simulink model "ClosedLoop"  (R2018b)
settings: Solver=VariableStepAuto  StartTime=0.0  StopTime=10  RelTol=1e-3
libraries: neural x533
(part 16 of 24)

== system ClosedLoop/Feed-Forward Neural Network/Layer 1/IW{1,1} ==
  "pd{1,1}" : Inport  PortDimensions=5
      mask Display: e = 0.06;c1 = [120 230 180]/255;c2 = ([120 230 180]+0)/(256+128);c3 = ([120 230 180]+128)/(256+128);patch([0 1 1 0],[0 0 1 1],c1);patch([0 1 1 1-e 1-e 0+e],[0 0 1 1-e 0+e 0+e],c2);patch([0 0 1 1-e 0+e 0+e],[0 1 1 1-e 1-e 0+e],c3);plot([0 1 1 0 0],[0 0 1 1 0]);
  "IW{1,1}(1,:)'" : Constant  Value=[0.777433677520860566545479741762392222881317138671875;0.73019317994989474396305695336195640265941619873046875;-0.69689232254614952299931474044569768011569976806640625;0.5351561132679254484401099034585058689117431640625;0.8471870111859789442831925043719820678234100341796875]
      mask Display: e = 0.06;c1 = [120 150 230]/255;c2 = ([120 150 230]+0)/383;c3 = ([120 150 230]+128)/383;patch([0 1 1 0],[0 0 1 1],c1);patch([0 1 1 1-e 1-e 0+e],[0 0 1 1-e 0+e 0+e],c2);patch([0 0 1 1-e 0+e 0+e],[0 1 1 1-e 1-e 0+e],c3);plot([0 1 1 0 0],[0 0 1 1 0]);disp('Weights');
  "IW{1,1}(10,:)'" : Constant  Value=[-0.08887973831498015286900482578857918269932270050048828125;-0.148128852319696802108950350884697400033473968505859375;0.489876132094335614564073466681293211877346038818359375;-0.004453902948160336737470910151159841916523873805999755859375;-0.36708303277551956877999828066094778478145599365234375]
      mask Display: e = 0.06;c1 = [120 150 230]/255;c2 = ([120 150 230]+0)/383;c3 = ([120 150 230]+128)/383;patch([0 1 1 0],[0 0 1 1],c1);patch([0 1 1 1-e 1-e 0+e],[0 0 1 1-e 0+e 0+e],c2);patch([0 0 1 1-e 0+e 0+e],[0 1 1 1-e 1-e 0+e],c3);plot([0 1 1 0 0],[0 0 1 1 0]);disp('Weights');
  "IW{1,1}(11,:)'" : Constant  Value=[0.257842561827505090121803732472471892833709716796875;0.2159497882699046578114376870871637947857379913330078125;-0.1732667109248870185300717139398329891264438629150390625;-0.229891953399321113948872152832336723804473876953125;-0.289081418236195986093406418149243108928203582763671875]
      mask Display: e = 0.06;c1 = [120 150 230]/255;c2 = ([120 150 230]+0)/383;c3 = ([120 150 230]+128)/383;patch([0 1 1 0],[0 0 1 1],c1);patch([0 1 1 1-e 1-e 0+e],[0 0 1 1-e 0+e 0+e],c2);patch([0 0 1 1-e 0+e 0+e],[0 1 1 1-e 1-e 0+e],c3);plot([0 1 1 0 0],[0 0 1 1 0]);disp('Weights');
  "IW{1,1}(12,:)'" : Constant  Value=[0.99297918861983658356251680743298493325710296630859375;-0.85768613628434042794879132998175919055938720703125;-0.1692019190082666157959323527393280528485774993896484375;-0.0360713330703844314850670116356923244893550872802734375;-0.82372546542318836326757036658818833529949188232421875]
      mask Display: e = 0.06;c1 = [120 150 230]/255;c2 = ([120 150 230]+0)/383;c3 = ([120 150 230]+128)/383;patch([0 1 1 0],[0 0 1 1],c1);patch([0 1 1 1-e 1-e 0+e],[0 0 1 1-e 0+e 0+e],c2);patch([0 0 1 1-e 0+e 0+e],[0 1 1 1-e 1-e 0+e],c3);plot([0 1 1 0 0],[0 0 1 1 0]);disp('Weights');
  "IW{1,1}(13,:)'" : Constant  Value=[-0.5601984423210086827538134457427076995372772216796875;0.8495448623663961473795325218816287815570831298828125;0.9142783166217982593337865182547830045223236083984375;-0.3151571944657833856950901463278569281101226806640625;-0.403790280453586003517330027534626424312591552734375]
      mask Display: e = 0.06;c1 = [120 150 230]/255;c2 = ([120 150 230]+0)/383;c3 = ([120 150 230]+128)/383;patch([0 1 1 0],[0 0 1 1],c1);patch([0 1 1 1-e 1-e 0+e],[0 0 1 1-e 0+e 0+e],c2);patch([0 0 1 1-e 0+e 0+e],[0 1 1 1-e 1-e 0+e],c3);plot([0 1 1 0 0],[0 0 1 1 0]);disp('Weights');
  "IW{1,1}(14,:)'" : Constant  Value=[-0.22742222534104128417453694055438973009586334228515625;0.287165266863248114237450181462918408215045928955078125;-0.2107887312575451865814812890675966627895832061767578125;0.384901355748308915405431207545916549861431121826171875;0.35264429343572889496982725177076645195484161376953125]
      mask Display: e = 0.06;c1 = [120 150 230]/255;c2 = ([120 150 230]+0)/383;c3 = ([120 150 230]+128)/383;patch([0 1 1 0],[0 0 1 1],c1);patch([0 1 1 1-e 1-e 0+e],[0 0 1 1-e 0+e 0+e],c2);patch([0 0 1 1-e 0+e 0+e],[0 1 1 1-e 1-e 0+e],c3);plot([0 1 1 0 0],[0 0 1 1 0]);disp('Weights');
  "IW{1,1}(15,:)'" : Constant  Value=[-0.4675162416237463869350676759495399892330169677734375;-0.791000664204850156835391317144967615604400634765625;0.203085187031351921405075700022280216217041015625;-0.2321122752203861328013090314925648272037506103515625;0.0023001892920386790564180046203546226024627685546875]
      mask Display: e = 0.06;c1 = [120 150 230]/255;c2 = ([120 150 230]+0)/383;c3 = ([120 150 230]+128)/383;patch([0 1 1 0],[0 0 1 1],c1);patch([0 1 1 1-e 1-e 0+e],[0 0 1 1-e 0+e 0+e],c2);patch([0 0 1 1-e 0+e 0+e],[0 1 1 1-e 1-e 0+e],c3);plot([0 1 1 0 0],[0 0 1 1 0]);disp('Weights');
  "IW{1,1}(16,:)'" : Constant  Value=[-0.370253147285887040940366432550945319235324859619140625;0.4026322235831856222176838855375535786151885986328125;0.454093022082059316613111832339200191199779510498046875;0.2183286697378135354785655408704769797623157501220703125;0.84167058255132121136199430111446417868137359619140625]
      mask Display: e = 0.06;c1 = [120 150 230]/255;c2 = ([120 150 230]+0)/383;c3 = ([120 150 230]+128)/383;patch([0 1 1 0],[0 0 1 1],c1);patch([0 1 1 1-e 1-e 0+e],[0 0 1 1-e 0+e 0+e],c2);patch([0 0 1 1-e 0+e 0+e],[0 1 1 1-e 1-e 0+e],c3);plot([0 1 1 0 0],[0 0 1 1 0]);disp('Weights');
  "IW{1,1}(17,:)'" : Constant  Value=[-0.6232209169783458069247217281372286379337310791015625;-0.208391342343335228548539816983975470066070556640625;0.357556683342926451274479404673911631107330322265625;-0.03813318521609776468039854080416262149810791015625;-0.8842941938241233312822942025377415120601654052734375]
      mask Display: e = 0.06;c1 = [120 150 230]/255;c2 = ([120 150 230]+0)/383;c3 = ([120 150 230]+128)/383;patch([0 1 1 0],[0 0 1 1],c1);patch([0 1 1 1-e 1-e 0+e],[0 0 1 1-e 0+e 0+e],c2);patch([0 0 1 1-e 0+e 0+e],[0 1 1 1-e 1-e 0+e],c3);plot([0 1 1 0 0],[0 0 1 1 0]);disp('Weights');
  "IW{1,1}(18,:)'" : Constant  Value=[-0.73987952043528881773681860067881643772125244140625;-0.82018478772733593995525325226481072604656219482421875;-0.3600533958394851463680197412031702697277069091796875;0.3501309983575382478449000700493343174457550048828125;-0.008329197715858167871960660022523370571434497833251953125]
      mask Display: e = 0.06;c1 = [120 150 230]/255;c2 = ([120 150 230]+0)/383;c3 = ([120 150 230]+128)/383;patch([0 1 1 0],[0 0 1 1],c1);patch([0 1 1 1-e 1-e 0+e],[0 0 1 1-e 0+e 0+e],c2);patch([0 0 1 1-e 0+e 0+e],[0 1 1 1-e 1-e 0+e],c3);plot([0 1 1 0 0],[0 0 1 1 0]);disp('Weights');
  "IW{1,1}(19,:)'" : Constant  Value=[-0.189399706316041804843308682393399067223072052001953125;-0.575158414122049155281501953140832483768463134765625;-0.64617497840545379261811831383965909481048583984375;0.61003694509276495949734453461132943630218505859375;-0.01759269567811309886717907602360355667769908905029296875]
      mask Display: e = 0.06;c1 = [120 150 230]/255;c2 = ([120 150 230]+0)/383;c3 = ([120 150 230]+128)/383;patch([0 1 1 0],[0 0 1 1],c1);patch([0 1 1 1-e 1-e 0+e],[0 0 1 1-e 0+e 0+e],c2);patch([0 0 1 1-e 0+e 0+e],[0 1 1 1-e 1-e 0+e],c3);plot([0 1 1 0 0],[0 0 1 1 0]);disp('Weights');
  "IW{1,1}(2,:)'" : Constant  Value=[0.63621458796631624732498266894253902137279510498046875;0.0583211436143939165877014829675317741930484771728515625;0.2549619279325689991111403287504799664020538330078125;-0.06918783634941839955079245783053920604288578033447265625;-0.52938238600419096346882952275336720049381256103515625]
      mask Display: e = 0.06;c1 = [120 150 230]/255;c2 = ([120 150 230]+0)/383;c3 = ([120 150 230]+128)/383;patch([0 1 1 0],[0 0 1 1],c1);patch([0 1 1 1-e 1-e 0+e],[0 0 1 1-e 0+e 0+e],c2);patch([0 0 1 1-e 0+e 0+e],[0 1 1 1-e 1-e 0+e],c3);plot([0 1 1 0 0],[0 0 1 1 0]);disp('Weights');
  "IW{1,1}(20,:)'" : Constant  Value=[-0.320099217953699832772684885640046559274196624755859375;-0.493413713263920694629405261366628110408782958984375;-0.258427516551161529090308022205135785043239593505859375;0.038020508091600242750462967933344771154224872589111328125;0.040457121285289963930065226804799749515950679779052734375]
      mask Display: e = 0.06;c1 = [120 150 230]/255;c2 = ([120 150 230]+0)/383;c3 = ([120 150 230]+128)/383;patch([0 1 1 0],[0 0 1 1],c1);patch([0 1 1 1-e 1-e 0+e],[0 0 1 1-e 0+e 0+e],c2);patch([0 0 1 1-e 0+e 0+e],[0 1 1 1-e 1-e 0+e],c3);plot([0 1 1 0 0],[0 0 1 1 0]);disp('Weights');
  "IW{1,1}(3,:)'" : Constant  Value=[-0.55562414003558036057484059710986912250518798828125;0.828270336283832175894303873064927756786346435546875;0.50830517043565492940615513361990451812744140625;-0.070744457945359773276550185983069241046905517578125;0.746438680345809846272686627344228327274322509765625]
      mask Display: e = 0.06;c1 = [120 150 230]/255;c2 = ([120 150 230]+0)/383;c3 = ([120 150 230]+128)/383;patch([0 1 1 0],[0 0 1 1],c1);patch([0 1 1 1-e 1-e 0+e],[0 0 1 1-e 0+e 0+e],c2);patch([0 0 1 1-e 0+e 0+e],[0 1 1 1-e 1-e 0+e],c3);plot([0 1 1 0 0],[0 0 1 1 0]);disp('Weights');
  "IW{1,1}(4,:)'" : Constant  Value=[0.75580233193780987921428504705545492470264434814453125;0.9364857196000182515405185768031515181064605712890625;-0.00704463179962803477673904950506766908802092075347900390625;-0.121740150618717624109166308699059300124645233154296875;-0.5242409013589768296270676728454418480396270751953125]
      mask Display: e = 0.06;c1 = [120 150 230]/255;c2 = ([120 150 230]+0)/383;c3 = ([120 150 230]+128)/383;patch([0 1 1 0],[0 0 1 1],c1);patch([0 1 1 1-e 1-e 0+e],[0 0 1 1-e 0+e 0+e],c2);patch([0 0 1 1-e 0+e 0+e],[0 1 1 1-e 1-e 0+e],c3);plot([0 1 1 0 0],[0 0 1 1 0]);disp('Weights');
  "IW{1,1}(5,:)'" : Constant  Value=[-1.233281510246877044068014583899639546871185302734375;0.1540174951845404149874951826859614811837673187255859375;0.3254058096269802913269586497335694730281829833984375;0.52623232596991720289025806778226979076862335205078125;0.15639372788910943512519224896095693111419677734375]
      mask Display: e = 0.06;c1 = [120 150 230]/255;c2 = ([120 150 230]+0)/383;c3 = ([120 150 230]+128)/383;patch([0 1 1 0],[0 0 1 1],c1);patch([0 1 1 1-e 1-e 0+e],[0 0 1 1-e 0+e 0+e],c2);patch([0 0 1 1-e 0+e 0+e],[0 1 1 1-e 1-e 0+e],c3);plot([0 1 1 0 0],[0 0 1 1 0]);disp('Weights');
  "IW{1,1}(6,:)'" : Constant  Value=[-0.2123808527301400961295740899004158563911914825439453125;-0.7650063601999883555748738217516802251338958740234375;0.2036265237720711607227741524184239096939563751220703125;0.2350543570458159259306540889156167395412921905517578125;-0.61247535013271681147983827031566761434078216552734375]
      mask Display: e = 0.06;c1 = [120 150 230]/255;c2 = ([120 150 230]+0)/383;c3 = ([120 150 230]+128)/383;patch([0 1 1 0],[0 0 1 1],c1);patch([0 1 1 1-e 1-e 0+e],[0 0 1 1-e 0+e 0+e],c2);patch([0 0 1 1-e 0+e 0+e],[0 1 1 1-e 1-e 0+e],c3);plot([0 1 1 0 0],[0 0 1 1 0]);disp('Weights');
  "IW{1,1}(7,:)'" : Constant  Value=[-0.145913693400883115458555039367638528347015380859375;0.85518026859664908467806299086078070104122161865234375;0.62282664130440179572900660787126980721950531005859375;0.2429637230793593172251121359295211732387542724609375;0.43881248529995386942204049773863516747951507568359375]
      mask Display: e = 0.06;c1 = [120 150 230]/255;c2 = ([120 150 230]+0)/383;c3 = ([120 150 230]+128)/383;patch([0 1 1 0],[0 0 1 1],c1);patch([0 1 1 1-e 1-e 0+e],[0 0 1 1-e 0+e 0+e],c2);patch([0 0 1 1-e 0+e 0+e],[0 1 1 1-e 1-e 0+e],c3);plot([0 1 1 0 0],[0 0 1 1 0]);disp('Weights');
  "IW{1,1}(8,:)'" : Constant  Value=[-0.19941423223278942344904862693510949611663818359375;0.1871215449623158111336351794307120144367218017578125;0.2685564059652356672103223900194279849529266357421875;-0.677958190830524554115754654048942029476165771484375;-0.6415809984175366853520472432137466967105865478515625]
      mask Display: e = 0.06;c1 = [120 150 230]/255;c2 = ([120 150 230]+0)/383;c3 = ([120 150 230]+128)/383;patch([0 1 1 0],[0 0 1 1],c1);patch([0 1 1 1-e 1-e 0+e],[0 0 1 1-e 0+e 0+e],c2);patch([0 0 1 1-e 0+e 0+e],[0 1 1 1-e 1-e 0+e],c3);plot([0 1 1 0 0],[0 0 1 1 0]);disp('Weights');
  "IW{1,1}(9,:)'" : Constant  Value=[-0.7761547121882117483693264148314483463764190673828125;0.767230609849536282496273997821845114231109619140625;0.20091122506164094119185392628423869609832763671875;-0.1352463461126560684277819746057502925395965576171875;-0.669215506292098805118939708336256444454193115234375]
      mask Display: e = 0.06;c1 = [120 150 230]/255;c2 = ([120 150 230]+0)/383;c3 = ([120 150 230]+128)/383;patch([0 1 1 0],[0 0 1 1],c1);patch([0 1 1 1-e 1-e 0+e],[0 0 1 1-e 0+e 0+e],c2);patch([0 0 1 1-e 0+e 0+e],[0 1 1 1-e 1-e 0+e],c3);plot([0 1 1 0 0],[0 0 1 1 0]);disp('Weights');
  Mux : Mux  Inputs=20
      mask Display: e = 0.06;c1 = [120 150 230]/255;c2 = ([120 150 230]+0)/383;c3 = ([120 150 230]+128)/383;patch([0 1 1 0],[0 0 1 1],c1);patch([0 1 1 1-e 1-e 0+e],[0 0 1 1-e 0+e 0+e],c2);patch([0 0 1 1-e 0+e 0+e],[0 1 1 1-e 1-e 0+e],c3);plot([0 1 1 0 0],[0 0 1 1 0]);disp('Mux');
  dotprod{1..20} (20 alike) : neural/Weight Functions/dotprod
  "iz{1,1}" : Outport
      mask Display: e = 0.06;c1 = [120 230 180]/255;c2 = ([120 230 180]+0)/(256+128);c3 = ([120 230 180]+128)/(256+128);patch([0 1 1 0],[0 0 1 1],c1);patch([0 1 1 1-e 1-e 0+e],[0 0 1 1-e 0+e 0+e],c2);patch([0 0 1 1-e 0+e 0+e],[0 1 1 1-e 1-e 0+e],c3);plot([0 1 1 0 0],[0 0 1 1 0]);
  wires:
  Mux/1 -> "iz{1,1}"/1
  dotprod20/1 -> Mux/20
  "IW{1,1}(20,:)'"/1 -> dotprod20/1
  dotprod19/1 -> Mux/19
  "IW{1,1}(19,:)'"/1 -> dotprod19/1
  dotprod18/1 -> Mux/18
  "IW{1,1}(18,:)'"/1 -> dotprod18/1
  dotprod17/1 -> Mux/17
  "IW{1,1}(17,:)'"/1 -> dotprod17/1
  dotprod16/1 -> Mux/16
  "IW{1,1}(16,:)'"/1 -> dotprod16/1
  dotprod15/1 -> Mux/15
  "IW{1,1}(15,:)'"/1 -> dotprod15/1
  dotprod14/1 -> Mux/14
  "IW{1,1}(14,:)'"/1 -> dotprod14/1
  dotprod13/1 -> Mux/13
  "IW{1,1}(13,:)'"/1 -> dotprod13/1
  dotprod12/1 -> Mux/12
  "IW{1,1}(12,:)'"/1 -> dotprod12/1
  dotprod11/1 -> Mux/11
  "IW{1,1}(11,:)'"/1 -> dotprod11/1
  dotprod10/1 -> Mux/10
  "IW{1,1}(10,:)'"/1 -> dotprod10/1
  dotprod9/1 -> Mux/9
  "IW{1,1}(9,:)'"/1 -> dotprod9/1
  dotprod8/1 -> Mux/8
  "IW{1,1}(8,:)'"/1 -> dotprod8/1
  dotprod7/1 -> Mux/7
  "IW{1,1}(7,:)'"/1 -> dotprod7/1
  dotprod6/1 -> Mux/6
  "IW{1,1}(6,:)'"/1 -> dotprod6/1
  dotprod5/1 -> Mux/5
  "IW{1,1}(5,:)'"/1 -> dotprod5/1
  dotprod4/1 -> Mux/4
  "IW{1,1}(4,:)'"/1 -> dotprod4/1
  dotprod3/1 -> Mux/3
  "IW{1,1}(3,:)'"/1 -> dotprod3/1
  dotprod2/1 -> Mux/2
  "IW{1,1}(2,:)'"/1 -> dotprod2/1
  dotprod1/1 -> Mux/1
  "pd{1,1}"/1 -> dotprod20/2, dotprod19/2, dotprod18/2, dotprod17/2, dotprod16/2, dotprod15/2, dotprod14/2, dotprod13/2, dotprod12/2, dotprod11/2, dotprod10/2, dotprod9/2, dotprod8/2, dotprod7/2, dotprod6/2, dotprod5/2, dotprod4/2, dotprod3/2, dotprod2/2, dotprod1/2
  "IW{1,1}(1,:)'"/1 -> dotprod1/1

== system ClosedLoop/Feed-Forward Neural Network/Layer 10/Delays 1 ==
  "p{10}" : Inport  PortDimensions=20
      mask Display: e = 0.06;c1 = [120 230 180]/255;c2 = ([120 230 180]+0)/(256+128);c3 = ([120 230 180]+128)/(256+128);patch([0 1 1 0],[0 0 1 1],c1);patch([0 1 1 1-e 1-e 0+e],[0 0 1 1-e 0+e 0+e],c2);patch([0 0 1 1-e 0+e 0+e],[0 1 1 1-e 1-e 0+e],c3);plot([0 1 1 0 0],[0 0 1 1 0]);
  mux : Mux  Inputs=1
      mask Display: e = 0.06;c1 = [120 150 230]/255;c2 = ([120 150 230]+0)/383;c3 = ([120 150 230]+128)/383;patch([0 1 1 0],[0 0 1 1],c1);patch([0 1 1 1-e 1-e 0+e],[0 0 1 1-e 0+e 0+e],c2);patch([0 0 1 1-e 0+e 0+e],[0 1 1 1-e 1-e 0+e],c3);plot([0 1 1 0 0],[0 0 1 1 0]);disp('Mux')
  "pd{10,9}" : Outport
      mask Display: e = 0.06;c1 = [120 230 180]/255;c2 = ([120 230 180]+0)/(256+128);c3 = ([120 230 180]+128)/(256+128);patch([0 1 1 0],[0 0 1 1],c1);patch([0 1 1 1-e 1-e 0+e],[0 0 1 1-e 0+e 0+e],c2);patch([0 0 1 1-e 0+e 0+e],[0 1 1 1-e 1-e 0+e],c3);plot([0 1 1 0 0],[0 0 1 1 0]);
  wires:
  mux/1 -> "pd{10,9}"/1
  "p{10}"/1 -> mux/1

== system ClosedLoop/Feed-Forward Neural Network/Layer 10/LW{10,9} ==
  "ad{10,9}" : Inport  PortDimensions=20
      mask Display: e = 0.06;c1 = [120 230 180]/255;c2 = ([120 230 180]+0)/(256+128);c3 = ([120 230 180]+128)/(256+128);patch([0 1 1 0],[0 0 1 1],c1);patch([0 1 1 1-e 1-e 0+e],[0 0 1 1-e 0+e 0+e],c2);patch([0 0 1 1-e 0+e 0+e],[0 1 1 1-e 1-e 0+e],c3);plot([0 1 1 0 0],[0 0 1 1 0]);
  "IW{10,9}(1,:)'" : Constant  Value=[0.5466415304082350434811132799950428307056427001953125;-0.8271711330800453065847932521137408912181854248046875;0.621717062498548411753063192008994519710540771484375;-0.7617361424174025064104398552444763481616973876953125;0.323400873829868817921351364930160343647003173828125;0.5870808725143337181151537151890806853771209716796875;0.331754437350670006168229519971646368503570556640625;-0.81908419253871667109478948987089097499847412109375;0.8565616368669726199414071743376553058624267578125;0.706184991822760732560482210828922688961029052734375;-0.450365553497307669061910928576253354549407958984375;0.161786684402280389605266464059241116046905517578125;0.03591585902579108591226031421683728694915771484375;0.6471253790508237901946131387376226484775543212890625;-0.941846360469744237065015113330446183681488037109375;0.7218375932220528756744215570506639778614044189453125;0.8760431144644991174885717555298469960689544677734375;-0.5388868782146196689808448354597203433513641357421875;-0.0040941045081634985791652070474810898303985595703125;-0.9809642025486418059898596766288392245769500732421875]
      mask Display: e = 0.06;c1 = [120 150 230]/255;c2 = ([120 150 230]+0)/383;c3 = ([120 150 230]+128)/383;patch([0 1 1 0],[0 0 1 1],c1);patch([0 1 1 1-e 1-e 0+e],[0 0 1 1-e 0+e 0+e],c2);patch([0 0 1 1-e 0+e 0+e],[0 1 1 1-e 1-e 0+e],c3);plot([0 1 1 0 0],[0 0 1 1 0]);disp('weights');
  "IW{10,9}(10,:)'" : Constant  Value=[0.189578467104812631305321701802313327789306640625;-0.1971505451331568015138628879867610521614551544189453125;-0.0938551633204507407270966723444871604442596435546875;-0.0355861505184178472660505576641298830509185791015625;0.3106286001380731409682312005315907299518585205078125;-0.54752969328460177056427937714033760130405426025390625;-0.457848112424283471000308054499328136444091796875;0.066724722426169780220561733585782349109649658203125;0.3399176553675749001826034145778976380825042724609375;1.007552250911837976588003584765829145908355712890625;0.265730037797317464320911994946072809398174285888671875;-0.897550681116356496858088576118461787700653076171875;0.8924950068454950979912609909661114215850830078125;-0.734025961733759668703669376554898917675018310546875;0.30825870376673292216906929752440191805362701416015625;0.6367403979295145344252659924677573144435882568359375;0.9993387589299149720289960896479897201061248779296875;0.72728658684421232383243705044151283800601959228515625;-0.006671055503067472615408295411043582134880125522613525390625;0.53220228209855668932704020335222594439983367919921875]
      mask Display: e = 0.06;c1 = [120 150 230]/255;c2 = ([120 150 230]+0)/383;c3 = ([120 150 230]+128)/383;patch([0 1 1 0],[0 0 1 1],c1);patch([0 1 1 1-e 1-e 0+e],[0 0 1 1-e 0+e 0+e],c2);patch([0 0 1 1-e 0+e 0+e],[0 1 1 1-e 1-e 0+e],c3);plot([0 1 1 0 0],[0 0 1 1 0]);disp('weights');
  "IW{10,9}(11,:)'" : Constant  Value=[-0.4022891319285617495182805214426480233669281005859375;-0.684681661104177496923739454359747469425201416015625;-0.210482527346528502931732873548753559589385986328125;-0.009164173785581652964538079686462879180908203125;0.1336869968563314525766827500774525105953216552734375;-0.8154908488996941429149956093169748783111572265625;-0.7225052276356740410534484908566810190677642822265625;0.0533294738522041011918872754904441535472869873046875;0.59118399932295506715718147461302578449249267578125;0.5589665429530852325257228585542179644107818603515625;-0.260620748059805951157841263921000063419342041015625;-0.609699818746113120226937098777852952480316162109375;-0.17887626676285517390851964592002332210540771484375;-0.915665165190061802746868124813772737979888916015625;-0.2142521711594704836301161776646040380001068115234375;-0.279113013475847271394059134763665497303009033203125;-0.7416473991930951914497427424066700041294097900390625;-0.6497481904034076993781354758539237082004547119140625;-0.3051031869474079005755129401222802698612213134765625;0.6723350544936492756420420846552588045597076416015625]
      mask Display: e = 0.06;c1 = [120 150 230]/255;c2 = ([120 150 230]+0)/383;c3 = ([120 150 230]+128)/383;patch([0 1 1 0],[0 0 1 1],c1);patch([0 1 1 1-e 1-e 0+e],[0 0 1 1-e 0+e 0+e],c2);patch([0 0 1 1-e 0+e 0+e],[0 1 1 1-e 1-e 0+e],c3);plot([0 1 1 0 0],[0 0 1 1 0]);disp('weights');
  "IW{10,9}(12,:)'" : Constant  Value=[0.472535423523304742854378446281771175563335418701171875;-0.11729833819846562092958919265583972446620464324951171875;0.923190603308829960127468439168296754360198974609375;-0.37303267056098388110285668517462909221649169921875;-0.99375627128259669262888564844615757465362548828125;-0.482768672816777044687341913231648504734039306640625;-0.62074958062280927162390753437648527324199676513671875;0.30989821754524171648625952002475969493389129638671875;-0.4549131499265310907276216312311589717864990234375;0.991655015662607386417448651627637445926666259765625;-0.29993544946830674735593902369146235287189483642578125;-0.32489154519676832766350571546354331076145172119140625;-0.9793327969276492961370195189374499022960662841796875;-0.1979220780648585087391211345675401389598846435546875;0.2415191975738621987801479917834512889385223388671875;0.003048136298864800863839263911359012126922607421875;-0.4132587115501944463602512769284658133983612060546875;0.74981073939471365452646978155826218426227569580078125;0.544121005652982159261910055647604167461395263671875;0.23469808525191437897916557631106115877628326416015625]
      mask Display: e = 0.06;c1 = [120 150 230]/255;c2 = ([120 150 230]+0)/383;c3 = ([120 150 230]+128)/383;patch([0 1 1 0],[0 0 1 1],c1);patch([0 1 1 1-e 1-e 0+e],[0 0 1 1-e 0+e 0+e],c2);patch([0 0 1 1-e 0+e 0+e],[0 1 1 1-e 1-e 0+e],c3);plot([0 1 1 0 0],[0 0 1 1 0]);disp('weights');
  "IW{10,9}(13,:)'" : Constant  Value=[-0.2790275991646777864474415764561854302883148193359375;0.1921087329921764563778197043575346469879150390625;-0.9836433950387455382724510855041444301605224609375;-0.3529980607903995259988505495130084455013275146484375;0.3027029619324619336140358427655883133411407470703125;0.805139324920179699773825632291845977306365966796875;-0.0121052133967480823883988705347292125225067138671875;0.293128861832891995931049677892588078975677490234375;-0.4321697413435654500091231966507621109485626220703125;-0.02489408541289872545121397706679999828338623046875;-0.117315079294827651068544582813046872615814208984375;0.2856668033102902626296781818382441997528076171875;-0.3798620054401198320448429512907750904560089111328125;0.1914153748986400227494186765397898852825164794921875;-0.500452529632526843528239623992703855037689208984375;0.4953482368724262396852964229765348136425018310546875;-0.0462412526256865685780894636991433799266815185546875;-0.4407344712191016977698154732934199273586273193359375;-0.42942652906107259269674614188261330127716064453125;-0.9986097920558434370974509874940849840641021728515625]
      mask Display: e = 0.06;c1 = [120 150 230]/255;c2 = ([120 150 230]+0)/383;c3 = ([120 150 230]+128)/383;patch([0 1 1 0],[0 0 1 1],c1);patch([0 1 1 1-e 1-e 0+e],[0 0 1 1-e 0+e 0+e],c2);patch([0 0 1 1-e 0+e 0+e],[0 1 1 1-e 1-e 0+e],c3);plot([0 1 1 0 0],[0 0 1 1 0]);disp('weights');
  "IW{10,9}(14,:)'" : Constant  Value=[0.4369190502101643058807667330256663262844085693359375;-0.355337007376919533641057569184340536594390869140625;-0.2031226207170384601141677194391377270221710205078125;0.8182026275036318185840400474262423813343048095703125;-0.3658053117802866349705936954705975949764251708984375;-0.565304022594878663454665002063848078250885009765625;-0.8268329782883065970366942565306089818477630615234375;-0.6163385354199117927009865525178611278533935546875;0.4345114997214183372165052787750028073787689208984375;-0.7440346798558070684492804502951912581920623779296875;0.0322476965290927619633976064505986869335174560546875;-0.565192144773778437638611649163067340850830078125;-0.689586324724370314243060420267283916473388671875;0.8393585927691102899217412414145655930042266845703125;0.4546934662228012680174060733406804502010345458984375;0.6636997613296118370129761387943290174007415771484375;-0.740835135518632892370760600897483527660369873046875;0.6989520026872793057037824837607331573963165283203125;0.6487934190964834701986774234683252871036529541015625;-0.497449739803909718460772637627087533473968505859375]
      mask Display: e = 0.06;c1 = [120 150 230]/255;c2 = ([120 150 230]+0)/383;c3 = ([120 150 230]+128)/383;patch([0 1 1 0],[0 0 1 1],c1);patch([0 1 1 1-e 1-e 0+e],[0 0 1 1-e 0+e 0+e],c2);patch([0 0 1 1-e 0+e 0+e],[0 1 1 1-e 1-e 0+e],c3);plot([0 1 1 0 0],[0 0 1 1 0]);disp('weights');
  "IW{10,9}(15,:)'" : Constant  Value=[0.81888617750407999285044979842496104538440704345703125;0.5025381956551642215202946317731402814388275146484375;-0.0244554521771054300671721648541279137134552001953125;-0.0993267520517020496839677434763871133327484130859375;-0.468132325571704033251307919272221624851226806640625;-0.09717765831892821726256670444854535162448883056640625;0.98966986014234514801302111663972027599811553955078125;0.7609751275066820586090443612192757427692413330078125;-0.6307257641354617749840372198377735912799835205078125;-0.1676228780207849045069679050357080996036529541015625;-0.3440258172026455785186271896236576139926910400390625;-0.7504227920973811638560846404288895428180694580078125;0.9881650804532176035621660048491321504116058349609375;-0.4124483755117100969300736323930323123931884765625;-0.49281764969508190521452206667163409292697906494140625;-0.2110580359176890130612491702777333557605743408203125;-0.5437530697986987515690771033405326306819915771484375;0.3556834622381674915203575437772087752819061279296875;-0.5514986314494745300862632575444877147674560546875;-0.1793520366655853293114120106110931374132633209228515625]
      mask Display: e = 0.06;c1 = [120 150 230]/255;c2 = ([120 150 230]+0)/383;c3 = ([120 150 230]+128)/383;patch([0 1 1 0],[0 0 1 1],c1);patch([0 1 1 1-e 1-e 0+e],[0 0 1 1-e 0+e 0+e],c2);patch([0 0 1 1-e 0+e 0+e],[0 1 1 1-e 1-e 0+e],c3);plot([0 1 1 0 0],[0 0 1 1 0]);disp('weights');
  "IW{10,9}(16,:)'" : Constant  Value=[-0.807261281547004383440935271210037171840667724609375;-0.69747664444503654213036725195706821978092193603515625;0.2362735258440535890400724383653141558170318603515625;0.4972716005811157469196359670604579150676727294921875;-0.0791035934022248365948826176463626325130462646484375;0.82826415173932266267087243249989114701747894287109375;-0.7461955501513630739651716794469393789768218994140625;-0.570484902244871694421135543962009251117706298828125;0.66740671729979794690734706819057464599609375;0.4379669677018591666950442231609486043453216552734375;-0.067320615611759115903822703330661170184612274169921875;0.92242108976409731280199366665328852832317352294921875;-0.0995215907740083505217398851527832448482513427734375;0.0900786848374106607906242061289958655834197998046875;-0.62719102872585763552848447943688370287418365478515625;-0.806727306236569408071090947487391531467437744140625;-0.63785591144042452782514374121092259883880615234375;-0.518744383210614667945037581375800073146820068359375;0.72428274486928712061484247897169552743434906005859375;-0.04536905795470470847963184723994345404207706451416015625]
      mask Display: e = 0.06;c1 = [120 150 230]/255;c2 = ([120 150 230]+0)/383;c3 = ([120 150 230]+128)/383;patch([0 1 1 0],[0 0 1 1],c1);patch([0 1 1 1-e 1-e 0+e],[0 0 1 1-e 0+e 0+e],c2);patch([0 0 1 1-e 0+e 0+e],[0 1 1 1-e 1-e 0+e],c3);plot([0 1 1 0 0],[0 0 1 1 0]);disp('weights');
  "IW{10,9}(17,:)'" : Constant  Value=[-0.079824662453312489329704249030328355729579925537109375;-0.50863162741843892522553005619556643068790435791015625;-0.8599800118631446554928743353229947388172149658203125;-0.6294933410241403404228321960545144975185394287109375;0.2463218798189050762204033162561245262622833251953125;-0.61285062671762446928624967767973430454730987548828125;-0.6803704001432462344922669217339716851711273193359375;-0.1774127237379981014697705177241005003452301025390625;-0.660669974241251178881384475971572101116180419921875;0.343070582710990279462492935635964386165142059326171875;-0.98323676721291730640217565451166592538356781005859375;-0.59245292930485338178669962871936149895191192626953125;0.0904365751746156742996163302450440824031829833984375;0.5633635565556909252649120389833115041255950927734375;-0.40518767328097304858403049365733750164508819580078125;-0.4692167703492871044801404423196800053119659423828125;0.3440311556339554766026367360609583556652069091796875;0.957117910618051848103959855507127940654754638671875;0.843549532473236052254605965572409331798553466796875;0.7310783118291774851371656041010282933712005615234375]
      mask Display: e = 0.06;c1 = [120 150 230]/255;c2 = ([120 150 230]+0)/383;c3 = ([120 150 230]+128)/383;patch([0 1 1 0],[0 0 1 1],c1);patch([0 1 1 1-e 1-e 0+e],[0 0 1 1-e 0+e 0+e],c2);patch([0 0 1 1-e 0+e 0+e],[0 1 1 1-e 1-e 0+e],c3);plot([0 1 1 0 0],[0 0 1 1 0]);disp('weights');
  "IW{10,9}(18,:)'" : Constant  Value=[-0.741994973924807066367748120683245360851287841796875;0.76531031300398344452418086802936159074306488037109375;-0.7146241606467922391487945787957869470119476318359375;-0.830155959148634270405864299391396343708038330078125;0.603706861411432260666742877219803631305694580078125;-0.1606720355925517207396069352398626506328582763671875;0.48859267651597704240629127525608055293560028076171875;-0.53859492966335509311903706475277431309223175048828125;0.906531353405531259426197721040807664394378662109375;0.7759681652601961854287537789787165820598602294921875;-0.6899583681930383516345273164915852248668670654296875;0.892110625991080041785608045756816864013671875;-0.4753364439368537031072037279955111443996429443359375;-0.3452009165545935065466665037092752754688262939453125;-0.418831082050324543519792541701463051140308380126953125;0.5838900251042142830470993430935777723789215087890625;-0.3484303194405888870477383534307591617107391357421875;-0.498105927839950890501086178119294345378875732421875;-0.607485742647509763258995008072815835475921630859375;-0.86925862322098990109253691116464324295520782470703125]
      mask Display: e = 0.06;c1 = [120 150 230]/255;c2 = ([120 150 230]+0)/383;c3 = ([120 150 230]+128)/383;patch([0 1 1 0],[0 0 1 1],c1);patch([0 1 1 1-e 1-e 0+e],[0 0 1 1-e 0+e 0+e],c2);patch([0 0 1 1-e 0+e 0+e],[0 1 1 1-e 1-e 0+e],c3);plot([0 1 1 0 0],[0 0 1 1 0]);disp('weights');
  "IW{10,9}(19,:)'" : Constant  Value=[0.38736835788324730511789084630436263978481292724609375;0.52891329205685211345411289585172198712825775146484375;0.3084532647244804248742866548127494752407073974609375;-0.5859415921437653995695882258587516844272613525390625;0.1223282385631441204765224028960801661014556884765625;0.2590331905913878518532555972342379391193389892578125;0.2544295394265023713131768090534023940563201904296875;-0.3702353880002842156926590178045444190502166748046875;0.4450960903678173874453705138876102864742279052734375;0.426338109566266776351284306656452827155590057373046875;-0.270300401170748993973091955922427587211132049560546875;0.32578454574266169085916544645442627370357513427734375;0.76508246916542699267438365495763719081878662109375;-0.8094744632637753678494618725380860269069671630859375;-0.77472824799972894727062566744280047714710235595703125;0.873721485200615877175778223318047821521759033203125;0.5811750549824659106690205589984543621540069580078125;0.25099601908891866486328581231646239757537841796875;-0.88025669091856995063238855436793528497219085693359375;-0.23714177163528316061302803063881583511829376220703125]
      mask Display: e = 0.06;c1 = [120 150 230]/255;c2 = ([120 150 230]+0)/383;c3 = ([120 150 230]+128)/383;patch([0 1 1 0],[0 0 1 1],c1);patch([0 1 1 1-e 1-e 0+e],[0 0 1 1-e 0+e 0+e],c2);patch([0 0 1 1-e 0+e 0+e],[0 1 1 1-e 1-e 0+e],c3);plot([0 1 1 0 0],[0 0 1 1 0]);disp('weights');
  "IW{10,9}(2,:)'" : Constant  Value=[0.31123060134378077723482647343189455568790435791015625;-0.11598795207237037885317221252989838831126689910888671875;-0.9031465636276241326640956685878336429595947265625;-0.9137257980716524397024613790563307702541351318359375;0.878426312741913850601349622593261301517486572265625;-0.46316276823649926708270641029230318963527679443359375;-0.47001936920430587019126278391922824084758758544921875;-0.85988252843962076354955570423044264316558837890625;0.0404389900613393304951159734628163278102874755859375;0.73223200057365700477163272807956673204898834228515625;-0.324586775588731890618277020621462725102901458740234375;0.206905879304431328247204646686441265046596527099609375;0.4256621081495055580745656698127277195453643798828125;-0.1456485391270645468608790906728245317935943603515625;0.427151520781819227234876734655699692666530609130859375;0.311896339067110783815905961091630160808563232421875;0.19449678910000756104636820964515209197998046875;0.304548084206509084292946454297634772956371307373046875;0.852464370597582732358432622277177870273590087890625;0.7279212226910936056611944877658970654010772705078125]
      mask Display: e = 0.06;c1 = [120 150 230]/255;c2 = ([120 150 230]+0)/383;c3 = ([120 150 230]+128)/383;patch([0 1 1 0],[0 0 1 1],c1);patch([0 1 1 1-e 1-e 0+e],[0 0 1 1-e 0+e 0+e],c2);patch([0 0 1 1-e 0+e 0+e],[0 1 1 1-e 1-e 0+e],c3);plot([0 1 1 0 0],[0 0 1 1 0]);disp('weights');
  "IW{10,9}(20,:)'" : Constant  Value=[0.6218941345983728385959921070025302469730377197265625;0.4764935207095664093657205739873461425304412841796875;-0.5633608101601839113214964527287520468235015869140625;0.1178313244835218487338579507195390760898590087890625;-0.950391819316425578989537825691513717174530029296875;0.1701798976749068492697603005581186152994632720947265625;-0.255211410172140829022424668437452055513858795166015625;-0.89931808742833563297125465396675281226634979248046875;-0.7315031942423522171026206706301309168338775634765625;0.11690383331813263001475178270993637852370738983154296875;0.5030808077341248907288218106259591877460479736328125;-0.57215287191730457294625011854805052280426025390625;-0.79387785618508122098546664346940815448760986328125;-0.11663477531182397939346628845669329166412353515625;-0.4591994970012169829942649812437593936920166015625;0.1365171766850858947606184301548637449741363525390625;0.0920278100907252483153797584236599504947662353515625;0.73124786617159742707627856361796148121356964111328125;0.033322833210528236824732317700181738473474979400634765625;-0.6459797732454202190410796902142465114593505859375]
      mask Display: e = 0.06;c1 = [120 150 230]/255;c2 = ([120 150 230]+0)/383;c3 = ([120 150 230]+128)/383;patch([0 1 1 0],[0 0 1 1],c1);patch([0 1 1 1-e 1-e 0+e],[0 0 1 1-e 0+e 0+e],c2);patch([0 0 1 1-e 0+e 0+e],[0 1 1 1-e 1-e 0+e],c3);plot([0 1 1 0 0],[0 0 1 1 0]);disp('weights');
  "IW{10,9}(3,:)'" : Constant  Value=[-0.02031602154059468368085816791790421120822429656982421875;0.039538332958086251645024589151944383047521114349365234375;-0.1705817246055880698207829482271336019039154052734375;-0.6688836378425844220174667498213239014148712158203125;-0.9195092514700846653141752540250308811664581298828125;0.64101413113088667738992398881237022578716278076171875;-0.2123219243529231581302241238518035970628261566162109375;0.0823701472827002290078013402307988144457340240478515625;-0.07174878378001636747285374440252780914306640625;0.176941434600180358405197011961718089878559112548828125;0.641158872283298375549520642380230128765106201171875;0.379413823597398280895731659256853163242340087890625;-0.48026194520168363766288166516460478305816650390625;0.8406893651913047715851234897854737937450408935546875;-0.7588351001593081068818946732790209352970123291015625;0.7130752026432418677615032720495946705341339111328125;0.975903935312047554617720379610545933246612548828125;-0.69556114013925773864599477747105993330478668212890625;-0.80700067769816918872294309039716608822345733642578125;0.688133933404440512049404787831008434295654296875]
      mask Display: e = 0.06;c1 = [120 150 230]/255;c2 = ([120 150 230]+0)/383;c3 = ([120 150 230]+128)/383;patch([0 1 1 0],[0 0 1 1],c1);patch([0 1 1 1-e 1-e 0+e],[0 0 1 1-e 0+e 0+e],c2);patch([0 0 1 1-e 0+e 0+e],[0 1 1 1-e 1-e 0+e],c3);plot([0 1 1 0 0],[0 0 1 1 0]);disp('weights');
  "IW{10,9}(4,:)'" : Constant  Value=[-0.243878720534027537691912357331602834165096282958984375;0.2053074047445965499836262324606650508940219879150390625;0.45097811081470506877622028696350753307342529296875;0.0222118072027239765731110310298390686511993408203125;-0.6726830018999148119718256566557101905345916748046875;0.466089669839742259949133540430921129882335662841796875;0.477903121225886684531047876589582301676273345947265625;0.793635623487578545365295212832279503345489501953125;0.04705945783433929108241500216536223888397216796875;-0.43775260993461728720177461582352407276630401611328125;-0.1194660680146172049287400795947178266942501068115234375;0.416988437363446706740433000959455966949462890625;-0.7706279880577551200104835515958257019519805908203125;0.05602431763753745741496459231711924076080322265625;-0.334725525373758270308854889663052745163440704345703125;-0.4581190683758273873849020674242638051509857177734375;0.5246970050505328497791879271971993148326873779296875;0.1906912809358017046879041345164296217262744903564453125;-0.66967161403699559940605468000285327434539794921875;0.4672495276460342239488454652018845081329345703125]
      mask Display: e = 0.06;c1 = [120 150 230]/255;c2 = ([120 150 230]+0)/383;c3 = ([120 150 230]+128)/383;patch([0 1 1 0],[0 0 1 1],c1);patch([0 1 1 1-e 1-e 0+e],[0 0 1 1-e 0+e 0+e],c2);patch([0 0 1 1-e 0+e 0+e],[0 1 1 1-e 1-e 0+e],c3);plot([0 1 1 0 0],[0 0 1 1 0]);disp('weights');
  "IW{10,9}(5,:)'" : Constant  Value=[0.312086021341554442631860410983790643513202667236328125;-0.5316311225021383979338907010969705879688262939453125;-0.72191197792878991634779595187865197658538818359375;0.7345360376959693127218997688032686710357666015625;-0.1237533116555358247978801955468952655792236328125;0.204826120903209396573174672084860503673553466796875;0.87040101830124994020110307246795855462551116943359375;-0.08853618153821131431246982401717104949057102203369140625;-0.326375785380894622988989794976077973842620849609375;-0.1549542207904054114120384610941982828080654144287109375;-0.836576164986852166549624598701484501361846923828125;-0.7050839398264019397544188905158080160617828369140625;0.099338993182101376078207977116107940673828125;0.7416692795617814137898449189378879964351654052734375;-0.1503446850666245449001934275656822137534618377685546875;0.791895559244191193926099003874696791172027587890625;-0.6287682627862880568869741182425059378147125244140625;0.89447227077628010949439385512960143387317657470703125;0.6528124529816861087994084300589747726917266845703125;-0.74579974084589506500009292722097598016262054443359375]
      mask Display: e = 0.06;c1 = [120 150 230]/255;c2 = ([120 150 230]+0)/383;c3 = ([120 150 230]+128)/383;patch([0 1 1 0],[0 0 1 1],c1);patch([0 1 1 1-e 1-e 0+e],[0 0 1 1-e 0+e 0+e],c2);patch([0 0 1 1-e 0+e 0+e],[0 1 1 1-e 1-e 0+e],c3);plot([0 1 1 0 0],[0 0 1 1 0]);disp('weights');
  "IW{10,9}(6,:)'" : Constant  Value=[-0.8112836774170393283611701917834579944610595703125;0.2037554318795340435599428019486367702484130859375;0.2651145183040057862200455929269082844257354736328125;0.5325214763621530789095004365663044154644012451171875;-0.34866479190794752440751835820265114307403564453125;-0.226099811727342281386654576635919511318206787109375;-0.0605618052668830397777810503612272441387176513671875;-0.80075063415624203599918473628349602222442626953125;-0.33524210374604113127361415536142885684967041015625;0.4033614816033506134118624686379916965961456298828125;0.7311687429574467156356831765151582658290863037109375;0.3145273117122184824978603501222096383571624755859375;-0.562196468330570464644324601977132260799407958984375;-0.294378378783245242544808206730522215366363525390625;0.25471369446024016980345550109632313251495361328125;-0.582419208255237297322537415311671793460845947265625;0.0335400112410704220877732950611971318721771240234375;-0.2740619400978372421917583778849802911281585693359375;-0.9627070303100626613712620383012108504772186279296875;0.1784631816817288108012462544138543307781219482421875]
      mask Display: e = 0.06;c1 = [120 150 230]/255;c2 = ([120 150 230]+0)/383;c3 = ([120 150 230]+128)/383;patch([0 1 1 0],[0 0 1 1],c1);patch([0 1 1 1-e 1-e 0+e],[0 0 1 1-e 0+e 0+e],c2);patch([0 0 1 1-e 0+e 0+e],[0 1 1 1-e 1-e 0+e],c3);plot([0 1 1 0 0],[0 0 1 1 0]);disp('weights');
  "IW{10,9}(7,:)'" : Constant  Value=[-0.6640547652893165064824643195606768131256103515625;-0.61815320030233100734307072343653999269008636474609375;-0.5063330851888461214826975265168584883213043212890625;-0.7300981514021891438659395134891383349895477294921875;-0.8201352753790744909423438002704642713069915771484375;-0.856338084438377666884889549692161381244659423828125;-0.30282752635680421082753355221939273178577423095703125;0.56993698806741421858390594934462569653987884521484375;0.97657576443709626090594611014239490032196044921875;-0.1915175403314524904541116256950772367417812347412109375;-0.20440822860577856356911752300220541656017303466796875;0.444185042316994682654041071145911701023578643798828125;-0.3756488315800565747082373491139151155948638916015625;-0.19969517695271310486759830382652580738067626953125;-0.28810456087325053697867360824602656066417694091796875;0.9283363604921166523098463585483841598033905029296875;0.28030419042139254059975428390316665172576904296875;-0.164744630885432064015816422397620044648647308349609375;0.451591316151048249860622263440745882689952850341796875;0.98006316459439302146705585982999764382839202880859375]
      mask Display: e = 0.06;c1 = [120 150 230]/255;c2 = ([120 150 230]+0)/383;c3 = ([120 150 230]+128)/383;patch([0 1 1 0],[0 0 1 1],c1);patch([0 1 1 1-e 1-e 0+e],[0 0 1 1-e 0+e 0+e],c2);patch([0 0 1 1-e 0+e 0+e],[0 1 1 1-e 1-e 0+e],c3);plot([0 1 1 0 0],[0 0 1 1 0]);disp('weights');
  "IW{10,9}(8,:)'" : Constant  Value=[0.38285888211369323297361688673845492303371429443359375;0.38708572624391968108881201260373927652835845947265625;0.679944546441566988193017095909453928470611572265625;-0.8701586447601095120063519061659462749958038330078125;0.6206392719932394275161868790746666491031646728515625;1.0111390951356893364021516390494070947170257568359375;-0.09922639634282741372128811008224147371947765350341796875;0.242846412117507959305129361382569186389446258544921875;-0.052566195399927462261757682426832616329193115234375;-0.86603585618607759055720407559419982135295867919921875;-0.65891996780142891854126219186582602560520172119140625;0.53799237993559290149647722500958479940891265869140625;0.946266165655015090152346601826138794422149658203125;0.1958457809948541683553457914968021214008331298828125;0.157856723781330254841037685764604248106479644775390625;-0.1712798239216652973482268862426280975341796875;0.737901801040307336876367116929031908512115478515625;0.87592985735321027274125071926391683518886566162109375;0.6369543859523065787442419605213217437267303466796875;0.7378889532225814118504558791755698621273040771484375]
      mask Display: e = 0.06;c1 = [120 150 230]/255;c2 = ([120 150 230]+0)/383;c3 = ([120 150 230]+128)/383;patch([0 1 1 0],[0 0 1 1],c1);patch([0 1 1 1-e 1-e 0+e],[0 0 1 1-e 0+e 0+e],c2);patch([0 0 1 1-e 0+e 0+e],[0 1 1 1-e 1-e 0+e],c3);plot([0 1 1 0 0],[0 0 1 1 0]);disp('weights');
  "IW{10,9}(9,:)'" : Constant  Value=[-0.291669006265933727917172291199676692485809326171875;0.396125998435526260887939997701323591172695159912109375;0.6733416465825570185188553296029567718505859375;0.3448899030878005422806609203689731657505035400390625;-0.2008820505961332880673353429301641881465911865234375;0.321961693960763739585928533415426500141620635986328125;-0.386560764580124061051691342072444967925548553466796875;-0.095271814798869147722371053532697260379791259765625;0.4937218757819916703510898514650762081146240234375;0.895923863179442836468524546944536268711090087890625;-0.99137476526075729577058837094227783381938934326171875;0.209820678085647915889211390094715170562267303466796875;-0.381619019010987159390424494631588459014892578125;0.8230358563336441779512142602470703423023223876953125;0.69233318081260197818238566469517536461353302001953125;-0.540869572272875576146589082782156765460968017578125;0.2002367390801269575462129068910144269466400146484375;-0.480247009056526064085801408509723842144012451171875;-0.7681351638744413623527407253277488052845001220703125;0.211526637835127206965779578240471892058849334716796875]
      mask Display: e = 0.06;c1 = [120 150 230]/255;c2 = ([120 150 230]+0)/383;c3 = ([120 150 230]+128)/383;patch([0 1 1 0],[0 0 1 1],c1);patch([0 1 1 1-e 1-e 0+e],[0 0 1 1-e 0+e 0+e],c2);patch([0 0 1 1-e 0+e 0+e],[0 1 1 1-e 1-e 0+e],c3);plot([0 1 1 0 0],[0 0 1 1 0]);disp('weights');
  Mux : Mux  Inputs=20
      mask Display: e = 0.06;c1 = [120 150 230]/255;c2 = ([120 150 230]+0)/383;c3 = ([120 150 230]+128)/383;patch([0 1 1 0],[0 0 1 1],c1);patch([0 1 1 1-e 1-e 0+e],[0 0 1 1-e 0+e 0+e],c2);patch([0 0 1 1-e 0+e 0+e],[0 1 1 1-e 1-e 0+e],c3);plot([0 1 1 0 0],[0 0 1 1 0]);disp('Mux');
  dotprod{1..20} (20 alike) : neural/Weight Functions/dotprod
  "lz{10,9}" : Outport
      mask Display: e = 0.06;c1 = [120 230 180]/255;c2 = ([120 230 180]+0)/(256+128);c3 = ([120 230 180]+128)/(256+128);patch([0 1 1 0],[0 0 1 1],c1);patch([0 1 1 1-e 1-e 0+e],[0 0 1 1-e 0+e 0+e],c2);patch([0 0 1 1-e 0+e 0+e],[0 1 1 1-e 1-e 0+e],c3);plot([0 1 1 0 0],[0 0 1 1 0]);
  wires:
  Mux/1 -> "lz{10,9}"/1
  dotprod20/1 -> Mux/20
  "IW{10,9}(20,:)'"/1 -> dotprod20/1
  dotprod19/1 -> Mux/19
  "IW{10,9}(19,:)'"/1 -> dotprod19/1
  dotprod18/1 -> Mux/18
  "IW{10,9}(18,:)'"/1 -> dotprod18/1
  dotprod17/1 -> Mux/17
  "IW{10,9}(17,:)'"/1 -> dotprod17/1
  dotprod16/1 -> Mux/16
  "IW{10,9}(16,:)'"/1 -> dotprod16/1
  dotprod15/1 -> Mux/15
  "IW{10,9}(15,:)'"/1 -> dotprod15/1
  dotprod14/1 -> Mux/14
  "IW{10,9}(14,:)'"/1 -> dotprod14/1
  dotprod13/1 -> Mux/13
  "IW{10,9}(13,:)'"/1 -> dotprod13/1
  dotprod12/1 -> Mux/12
  "IW{10,9}(12,:)'"/1 -> dotprod12/1
  dotprod11/1 -> Mux/11
  "IW{10,9}(11,:)'"/1 -> dotprod11/1
  dotprod10/1 -> Mux/10
  "IW{10,9}(10,:)'"/1 -> dotprod10/1
  dotprod9/1 -> Mux/9
  "IW{10,9}(9,:)'"/1 -> dotprod9/1
  dotprod8/1 -> Mux/8
  "IW{10,9}(8,:)'"/1 -> dotprod8/1
  dotprod7/1 -> Mux/7
  "IW{10,9}(7,:)'"/1 -> dotprod7/1
  dotprod6/1 -> Mux/6
  "IW{10,9}(6,:)'"/1 -> dotprod6/1
  dotprod5/1 -> Mux/5
  "IW{10,9}(5,:)'"/1 -> dotprod5/1
  dotprod4/1 -> Mux/4
  "IW{10,9}(4,:)'"/1 -> dotprod4/1
  dotprod3/1 -> Mux/3
  "IW{10,9}(3,:)'"/1 -> dotprod3/1
  dotprod2/1 -> Mux/2
  "IW{10,9}(2,:)'"/1 -> dotprod2/1
  dotprod1/1 -> Mux/1
  "ad{10,9}"/1 -> dotprod20/2, dotprod19/2, dotprod18/2, dotprod17/2, dotprod16/2, dotprod15/2, dotprod14/2, dotprod13/2, dotprod12/2, dotprod11/2, dotprod10/2, dotprod9/2, dotprod8/2, dotprod7/2, dotprod6/2, dotprod5/2, dotprod4/2, dotprod3/2, dotprod2/2, dotprod1/2
  "IW{10,9}(1,:)'"/1 -> dotprod1/1

== system ClosedLoop/Feed-Forward Neural Network/Layer 11/Delays 1 ==
  "p{11}" : Inport  PortDimensions=20
      mask Display: e = 0.06;c1 = [120 230 180]/255;c2 = ([120 230 180]+0)/(256+128);c3 = ([120 230 180]+128)/(256+128);patch([0 1 1 0],[0 0 1 1],c1);patch([0 1 1 1-e 1-e 0+e],[0 0 1 1-e 0+e 0+e],c2);patch([0 0 1 1-e 0+e 0+e],[0 1 1 1-e 1-e 0+e],c3);plot([0 1 1 0 0],[0 0 1 1 0]);
  mux : Mux  Inputs=1
      mask Display: e = 0.06;c1 = [120 150 230]/255;c2 = ([120 150 230]+0)/383;c3 = ([120 150 230]+128)/383;patch([0 1 1 0],[0 0 1 1],c1);patch([0 1 1 1-e 1-e 0+e],[0 0 1 1-e 0+e 0+e],c2);patch([0 0 1 1-e 0+e 0+e],[0 1 1 1-e 1-e 0+e],c3);plot([0 1 1 0 0],[0 0 1 1 0]);disp('Mux')
  "pd{11,10}" : Outport
      mask Display: e = 0.06;c1 = [120 230 180]/255;c2 = ([120 230 180]+0)/(256+128);c3 = ([120 230 180]+128)/(256+128);patch([0 1 1 0],[0 0 1 1],c1);patch([0 1 1 1-e 1-e 0+e],[0 0 1 1-e 0+e 0+e],c2);patch([0 0 1 1-e 0+e 0+e],[0 1 1 1-e 1-e 0+e],c3);plot([0 1 1 0 0],[0 0 1 1 0]);
  wires:
  mux/1 -> "pd{11,10}"/1
  "p{11}"/1 -> mux/1
